simulink model "MR30Simulinknodos"  (R2013a)
settings: Solver=ode23tb  StartTime=0.0  StopTime=10.0  RelTol=1e-3
libraries: powerlib x200
(part 2 of 2)

== system MR30Simulinknodos/BUSstep B25 ==
  " (RL1)/2" : powerlib/Elements/Series RLC Branch  LConnTagsString=__new0  RConnTagsString=__new0  BranchType=R  Resistance=1.560804/2  Inductance=1e-3  SetiL0=off  InitialCurrent=0  Capacitance=1e-6  Setx0=off  InitialVoltage=0  Measurements=None
  " (RL3)/2" : powerlib/Elements/Series RLC Branch  LConnTagsString=__new0  RConnTagsString=__new0  BranchType=R  Resistance=3.632832/2  Inductance=1e-3  SetiL0=off  InitialCurrent=0  Capacitance=1e-6  Setx0=off  InitialVoltage=0  Measurements=None
  " (RLn)/2" : powerlib/Elements/Series RLC Branch  LConnTagsString=__new0  RConnTagsString=__new0  BranchType=R  Resistance=2.69178/2  Inductance=1e-3  SetiL0=off  InitialCurrent=0  Capacitance=1e-6  Setx0=off  InitialVoltage=0  Measurements=None
  Ground : powerlib/Elements/Ground  LConnTagsString=a
  Voltage Measurement : powerlib/Measurements/Voltage Measurement  PhasorSimulation=off  OutputType=Complex  PSBequivalent=0
  L35 : PMIOPort  Port=1  Side=Right
  L34 : PMIOPort  Port=2  Side=Right
  L33 : PMIOPort  Port=3  Side=Left
  VBUSstep : Outport
  wires:
  Voltage Measurement/1 -> VBUSstep/1
  connections:
  L33/RConn1 -- " (RLn)/2"/RConn1
  " (RL3)/2"/RConn1 -- " (RLn)/2"/LConn1 -- " (RL1)/2"/LConn1 -- Voltage Measurement/LConn1
  Ground/LConn1 -- Voltage Measurement/LConn2
  " (RL3)/2"/LConn1 -- L34/RConn1
  " (RL1)/2"/RConn1 -- L35/RConn1

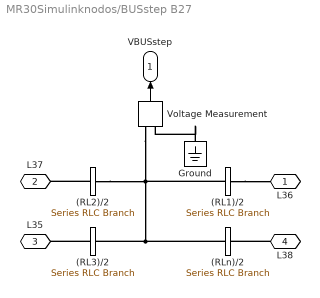
== system MR30Simulinknodos/BUSstep B27 ==
  " (RL1)/2" : powerlib/Elements/Series RLC Branch  LConnTagsString=__new0  RConnTagsString=__new0  BranchType=R  Resistance=5.65488/2  Inductance=1e-3  SetiL0=off  InitialCurrent=0  Capacitance=1e-6  Setx0=off  InitialVoltage=0  Measurements=None
  " (RL2)/2" : powerlib/Elements/Series RLC Branch  LConnTagsString=__new0  RConnTagsString=__new0  BranchType=R  Resistance=3.138744/2  Inductance=1e-3  SetiL0=off  InitialCurrent=0  Capacitance=1e-6  Setx0=off  InitialVoltage=0  Measurements=None
  " (RL3)/2" : powerlib/Elements/Series RLC Branch  LConnTagsString=__new0  RConnTagsString=__new0  BranchType=R  Resistance=1.560804/2  Inductance=1e-3  SetiL0=off  InitialCurrent=0  Capacitance=1e-6  Setx0=off  InitialVoltage=0  Measurements=None
  " (RLn)/2" : powerlib/Elements/Series RLC Branch  LConnTagsString=__new0  RConnTagsString=__new0  BranchType=R  Resistance=4.572456/2  Inductance=1e-3  SetiL0=off  InitialCurrent=0  Capacitance=1e-6  Setx0=off  InitialVoltage=0  Measurements=None
  Ground : powerlib/Elements/Ground  LConnTagsString=a
  Voltage Measurement : powerlib/Measurements/Voltage Measurement  PhasorSimulation=off  OutputType=Complex  PSBequivalent=0
  L36 : PMIOPort  Port=1  Side=Right
  L37 : PMIOPort  Port=2  Side=Left
  L35 : PMIOPort  Port=3  Side=Right
  L38 : PMIOPort  Port=4  Side=Left
  VBUSstep : Outport
  wires:
  Voltage Measurement/1 -> VBUSstep/1
  connections:
  " (RL1)/2"/RConn1 -- L36/RConn1
  " (RL3)/2"/LConn1 -- L35/RConn1
  " (RL2)/2"/LConn1 -- L37/RConn1
  Ground/LConn1 -- Voltage Measurement/LConn2
  Voltage Measurement/LConn1 -- " (RL2)/2"/RConn1 -- " (RL1)/2"/LConn1 -- " (RLn)/2"/LConn1 -- " (RL3)/2"/RConn1
  L38/RConn1 -- " (RLn)/2"/RConn1

== system MR30Simulinknodos/BUSstep B28 ==
  " (RL1)/2" : powerlib/Elements/Series RLC Branch  LConnTagsString=__new0  RConnTagsString=__new0  BranchType=R  Resistance=0.908208/2  Inductance=1e-3  SetiL0=off  InitialCurrent=0  Capacitance=1e-6  Setx0=off  InitialVoltage=0  Measurements=None
  " (RL2)/2" : powerlib/Elements/Series RLC Branch  LConnTagsString=__new0  RConnTagsString=__new0  BranchType=R  Resistance=5.65488/2  Inductance=1e-3  SetiL0=off  InitialCurrent=0  Capacitance=1e-6  Setx0=off  InitialVoltage=0  Measurements=None
  " (RL3)/2" : powerlib/Elements/Series RLC Branch  LConnTagsString=__new0  RConnTagsString=__new0  BranchType=R  Resistance=2.41332/2  Inductance=1e-3  SetiL0=off  InitialCurrent=0  Capacitance=1e-6  Setx0=off  InitialVoltage=0  Measurements=None
  Ground : powerlib/Elements/Ground  LConnTagsString=a
  Voltage Measurement : powerlib/Measurements/Voltage Measurement  PhasorSimulation=off  OutputType=Complex  PSBequivalent=0
  L40 : PMIOPort  Port=1  Side=Right
  L36 : PMIOPort  Port=2  Side=Left
  L41 : PMIOPort  Port=3  Side=Right
  VBUSstep : Outport
  wires:
  Voltage Measurement/1 -> VBUSstep/1
  connections:
  " (RL3)/2"/RConn1 -- " (RL1)/2"/LConn1 -- " (RL2)/2"/RConn1 -- Voltage Measurement/LConn1
  Ground/LConn1 -- Voltage Measurement/LConn2
  " (RL2)/2"/LConn1 -- L36/RConn1
  " (RL3)/2"/LConn1 -- L41/RConn1
  " (RL1)/2"/RConn1 -- L40/RConn1

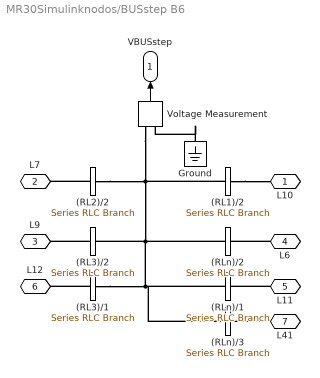
== system MR30Simulinknodos/BUSstep B6 ==
  " (RL1)/2" : powerlib/Elements/Series RLC Branch  LConnTagsString=__new0  RConnTagsString=__new0  BranchType=R  Resistance=.17136/2  Inductance=1e-3  SetiL0=off  InitialCurrent=0  Capacitance=1e-6  Setx0=off  InitialVoltage=0  Measurements=None
  " (RL2)/2" : powerlib/Elements/Series RLC Branch  LConnTagsString=__new0  RConnTagsString=__new0  BranchType=R  Resistance=0.169932/2  Inductance=1e-3  SetiL0=off  InitialCurrent=0  Capacitance=1e-6  Setx0=off  InitialVoltage=0  Measurements=None
  " (RL3)/1" : powerlib/Elements/Series RLC Branch  LConnTagsString=__new0  RConnTagsString=__new0  BranchType=R  Resistance=7.93968/2  Inductance=1e-3  SetiL0=off  InitialCurrent=0  Capacitance=1e-6  Setx0=off  InitialVoltage=0  Measurements=None
  " (RL3)/2" : powerlib/Elements/Series RLC Branch  LConnTagsString=__new0  RConnTagsString=__new0  BranchType=R  Resistance=.381276/2  Inductance=1e-3  SetiL0=off  InitialCurrent=0  Capacitance=1e-6  Setx0=off  InitialVoltage=0  Measurements=None
  " (RLn)/1" : powerlib/Elements/Series RLC Branch  LConnTagsString=__new0  RConnTagsString=__new0  BranchType=R  Resistance=2.97024/2  Inductance=1e-3  SetiL0=off  InitialCurrent=0  Capacitance=1e-6  Setx0=off  InitialVoltage=0  Measurements=None
  " (RLn)/2" : powerlib/Elements/Series RLC Branch  LConnTagsString=__new0  RConnTagsString=__new0  BranchType=R  Resistance=.829668/2  Inductance=1e-3  SetiL0=off  InitialCurrent=0  Capacitance=1e-6  Setx0=off  InitialVoltage=0  Measurements=None
  " (RLn)/3" : powerlib/Elements/Series RLC Branch  LConnTagsString=__new0  RConnTagsString=__new0  BranchType=R  Resistance=2.41332/2  Inductance=1e-3  SetiL0=off  InitialCurrent=0  Capacitance=1e-6  Setx0=off  InitialVoltage=0  Measurements=None
  Ground : powerlib/Elements/Ground  LConnTagsString=a
  Voltage Measurement : powerlib/Measurements/Voltage Measurement  PhasorSimulation=off  OutputType=Complex  PSBequivalent=0
  L10 : PMIOPort  Port=1  Side=Right
  L7 : PMIOPort  Port=2  Side=Left
  L9 : PMIOPort  Port=3  Side=Right
  L6 : PMIOPort  Port=4  Side=Left
  L11 : PMIOPort  Port=5  Side=Left
  L12 : PMIOPort  Port=6  Side=Right
  L41 : PMIOPort  Port=7  Side=Left
  VBUSstep : Outport
  wires:
  Voltage Measurement/1 -> VBUSstep/1
  connections:
  " (RL1)/2"/RConn1 -- L10/RConn1
  " (RL3)/2"/LConn1 -- L9/RConn1
  " (RL2)/2"/LConn1 -- L7/RConn1
  Ground/LConn1 -- Voltage Measurement/LConn2
  Voltage Measurement/LConn1 -- " (RL2)/2"/RConn1 -- " (RL1)/2"/LConn1 -- " (RLn)/3"/LConn1 -- " (RLn)/1"/LConn1 -- " (RL3)/1"/RConn1 -- " (RLn)/2"/LConn1 -- " (RL3)/2"/RConn1
  L6/RConn1 -- " (RLn)/2"/RConn1
  L11/RConn1 -- " (RLn)/1"/RConn1
  " (RL3)/1"/LConn1 -- L12/RConn1
  L41/RConn1 -- " (RLn)/3"/RConn1

== system MR30Simulinknodos/BUSstep B9 ==
  " (RL1)/2" : powerlib/Elements/Series RLC Branch  LConnTagsString=__new0  RConnTagsString=__new0  BranchType=R  Resistance=1.5708/2  Inductance=1e-3  SetiL0=off  InitialCurrent=0  Capacitance=1e-6  Setx0=off  InitialVoltage=0  Measurements=None
  " (RL2)/2" : powerlib/Elements/Series RLC Branch  LConnTagsString=__new0  RConnTagsString=__new0  BranchType=R  Resistance=2.97024/2  Inductance=1e-3  SetiL0=off  InitialCurrent=0  Capacitance=1e-6  Setx0=off  InitialVoltage=0  Measurements=None
  " (RLn)/2" : powerlib/Elements/Series RLC Branch  LConnTagsString=__new0  RConnTagsString=__new0  BranchType=R  Resistance=2.97024/2  Inductance=1e-3  SetiL0=off  InitialCurrent=0  Capacitance=1e-6  Setx0=off  InitialVoltage=0  Measurements=None
  Ground : powerlib/Elements/Ground  LConnTagsString=a
  Voltage Measurement : powerlib/Measurements/Voltage Measurement  PhasorSimulation=off  OutputType=Complex  PSBequivalent=0
  L14 : PMIOPort  Port=1  Side=Right
  L13 : PMIOPort  Port=2  Side=Left
  L11 : PMIOPort  Port=3  Side=Left
  VBUSstep : Outport
  wires:
  Voltage Measurement/1 -> VBUSstep/1
  connections:
  L11/RConn1 -- " (RLn)/2"/RConn1
  " (RLn)/2"/LConn1 -- " (RL1)/2"/LConn1 -- " (RL2)/2"/RConn1 -- Voltage Measurement/LConn1
  Ground/LConn1 -- Voltage Measurement/LConn2
  " (RL2)/2"/LConn1 -- L13/RConn1
  " (RL1)/2"/RConn1 -- L14/RConn1

== system MR30Simulinknodos/DG1 ==
  VBUS1 : Inport
  IBUS1 : Inport  Port=2
  DroopDG1 : Subsystem
  G1 : powerlib/Electrical Sources/Controlled Voltage Source  Initialize=on  Source_Type=DC  Amplitude=1000  Phase=0  Frequency=0  Measurements=None
  Ground : powerlib/Elements/Ground  LConnTagsString=a
  DG1+ : PMIOPort  Port=1  Side=Right
  DG1- : PMIOPort  Port=2  Side=Right
  PBUS1 : Outport
  wires:
  DroopDG1/2(PDG1) -> PBUS1/1
  IBUS1/1 -> DroopDG1/2(IG1)
  VBUS1/1 -> DroopDG1/1(VG1)
  DroopDG1/1(Vdroop1) -> G1/1
  connections:
  G1/LConn1 -- DG1-/RConn1 -- Ground/LConn1
  DG1+/RConn1 -- G1/RConn1

== system MR30Simulinknodos/DG2 ==
  VBUS2 : Inport
  IBUS2 : Inport  Port=2
  DroopDG1 : Subsystem
  G1 : powerlib/Electrical Sources/Controlled Voltage Source  Initialize=on  Source_Type=DC  Amplitude=1000  Phase=0  Frequency=0  Measurements=None
  Ground : powerlib/Elements/Ground  LConnTagsString=a
  DG2+ : PMIOPort  Port=1  Side=Right
  DG2- : PMIOPort  Port=2  Side=Right
  PBUS2 : Outport
  wires:
  VBUS2/1 -> DroopDG1/1(VG1)
  IBUS2/1 -> DroopDG1/2(IG1)
  DroopDG1/2(PDG1) -> PBUS2/1
  DroopDG1/1(Vdroop1) -> G1/1
  connections:
  DG2+/RConn1 -- G1/RConn1
  Ground/LConn1 -- DG2-/RConn1 -- G1/LConn1

== system MR30Simulinknodos/DG3 ==
  VBUS5 : Inport
  IBUS5 : Inport  Port=2
  DroopDG1 : Subsystem
  G1 : powerlib/Electrical Sources/Controlled Voltage Source  Initialize=on  Source_Type=DC  Amplitude=1000  Phase=0  Frequency=0  Measurements=None
  Ground : powerlib/Elements/Ground  LConnTagsString=a
  DG3+ : PMIOPort  Port=1  Side=Right
  DG3- : PMIOPort  Port=2  Side=Right
  PBUS5 : Outport
  wires:
  DroopDG1/2(PDG1) -> PBUS5/1
  IBUS5/1 -> DroopDG1/2(IG1)
  VBUS5/1 -> DroopDG1/1(VG1)
  DroopDG1/1(Vdroop1) -> G1/1
  connections:
  G1/LConn1 -- DG3-/RConn1 -- Ground/LConn1
  DG3+/RConn1 -- G1/RConn1

== system MR30Simulinknodos/DG4 ==
  VBUS8 : Inport
  IBUS8 : Inport  Port=2
  DroopDG1 : Subsystem
  G1 : powerlib/Electrical Sources/Controlled Voltage Source  Initialize=on  Source_Type=DC  Amplitude=1000  Phase=0  Frequency=0  Measurements=None
  Ground : powerlib/Elements/Ground  LConnTagsString=a
  DG4+ : PMIOPort  Port=1  Side=Right
  DG4- : PMIOPort  Port=2  Side=Right
  PBUS8 : Outport
  wires:
  VBUS8/1 -> DroopDG1/1(VG1)
  IBUS8/1 -> DroopDG1/2(IG1)
  DroopDG1/2(PDG1) -> PBUS8/1
  DroopDG1/1(Vdroop1) -> G1/1
  connections:
  DG4+/RConn1 -- G1/RConn1
  Ground/LConn1 -- DG4-/RConn1 -- G1/LConn1

== system MR30Simulinknodos/DG5 ==
  VBUS11 : Inport
  IBUS11 : Inport  Port=2
  DroopDG1 : Subsystem
  G1 : powerlib/Electrical Sources/Controlled Voltage Source  Initialize=on  Source_Type=DC  Amplitude=1000  Phase=0  Frequency=0  Measurements=None
  Ground : powerlib/Elements/Ground  LConnTagsString=a
  DG5+ : PMIOPort  Port=1  Side=Right
  DG5- : PMIOPort  Port=2  Side=Right
  PBUS11 : Outport
  wires:
  VBUS11/1 -> DroopDG1/1(VG1)
  IBUS11/1 -> DroopDG1/2(IG1)
  DroopDG1/2(PDG1) -> PBUS11/1
  DroopDG1/1(Vdroop1) -> G1/1
  connections:
  DG5+/RConn1 -- G1/RConn1
  Ground/LConn1 -- DG5-/RConn1 -- G1/LConn1

== system MR30Simulinknodos/DG6 ==
  VBUS13 : Inport
  IBUS13 : Inport  Port=2
  DroopDG1 : Subsystem
  G1 : powerlib/Electrical Sources/Controlled Voltage Source  Initialize=on  Source_Type=DC  Amplitude=1000  Phase=0  Frequency=0  Measurements=None
  Ground : powerlib/Elements/Ground  LConnTagsString=a
  DG6+ : PMIOPort  Port=1  Side=Right
  DG6- : PMIOPort  Port=2  Side=Right
  PBUS13 : Outport
  wires:
  DroopDG1/2(PDG1) -> PBUS13/1
  IBUS13/1 -> DroopDG1/2(IG1)
  VBUS13/1 -> DroopDG1/1(VG1)
  DroopDG1/1(Vdroop1) -> G1/1
  connections:
  G1/LConn1 -- DG6-/RConn1 -- Ground/LConn1
  DG6+/RConn1 -- G1/RConn1

== system MR30Simulinknodos/Load1 ==
  VBUSc : Inport
  Constant4 : Constant  Value=21700
  Controlled Current Source : powerlib/Electrical Sources/Controlled Current Source  Initialize=off  Source_Type=DC  Amplitude=0  Phase=0  Frequency=0  Measurements=None
  Divide2 : Product  Inputs=*/
  Ground3 : powerlib/Elements/Ground  LConnTagsString=a
  Load1+ : PMIOPort  Port=1  Side=Left
  Load1- : PMIOPort  Port=2  Side=Left
  wires:
  Constant4/1 -> Divide2/1
  Divide2/1 -> Controlled Current Source/1
  VBUSc/1 -> Divide2/2
  connections:
  Controlled Current Source/RConn1 -- Load1-/RConn1 -- Ground3/LConn1
  Controlled Current Source/LConn1 -- Load1+/RConn1

== system MR30Simulinknodos/Load10 ==
  VBUSc : Inport
  Constant4 : Constant  Value=8200
  Controlled Current Source : powerlib/Electrical Sources/Controlled Current Source  Initialize=off  Source_Type=DC  Amplitude=0  Phase=0  Frequency=0  Measurements=None
  Divide2 : Product  Inputs=*/
  Ground3 : powerlib/Elements/Ground  LConnTagsString=a
  Load1+ : PMIOPort  Port=1  Side=Left
  Load1- : PMIOPort  Port=2  Side=Left
  wires:
  VBUSc/1 -> Divide2/2
  Divide2/1 -> Controlled Current Source/1
  Constant4/1 -> Divide2/1
  connections:
  Controlled Current Source/LConn1 -- Load1+/RConn1
  Ground3/LConn1 -- Load1-/RConn1 -- Controlled Current Source/RConn1

== system MR30Simulinknodos/Load11 ==
  VBUSc : Inport
  Constant4 : Constant  Value=3500
  Controlled Current Source : powerlib/Electrical Sources/Controlled Current Source  Initialize=off  Source_Type=DC  Amplitude=0  Phase=0  Frequency=0  Measurements=None
  Divide2 : Product  Inputs=*/
  Ground3 : powerlib/Elements/Ground  LConnTagsString=a
  Load1+ : PMIOPort  Port=1  Side=Left
  Load1- : PMIOPort  Port=2  Side=Left
  wires:
  Constant4/1 -> Divide2/1
  Divide2/1 -> Controlled Current Source/1
  VBUSc/1 -> Divide2/2
  connections:
  Controlled Current Source/RConn1 -- Load1-/RConn1 -- Ground3/LConn1
  Controlled Current Source/LConn1 -- Load1+/RConn1

== system MR30Simulinknodos/Load12 ==
  VBUSc : Inport
  Constant4 : Constant  Value=9000
  Controlled Current Source : powerlib/Electrical Sources/Controlled Current Source  Initialize=off  Source_Type=DC  Amplitude=0  Phase=0  Frequency=0  Measurements=None
  Divide2 : Product  Inputs=*/
  Ground3 : powerlib/Elements/Ground  LConnTagsString=a
  Load1+ : PMIOPort  Port=1  Side=Left
  Load1- : PMIOPort  Port=2  Side=Left
  wires:
  VBUSc/1 -> Divide2/2
  Divide2/1 -> Controlled Current Source/1
  Constant4/1 -> Divide2/1
  connections:
  Controlled Current Source/LConn1 -- Load1+/RConn1
  Ground3/LConn1 -- Load1-/RConn1 -- Controlled Current Source/RConn1

== system MR30Simulinknodos/Load13 ==
  VBUSc : Inport
  Constant4 : Constant  Value=3200
  Controlled Current Source : powerlib/Electrical Sources/Controlled Current Source  Initialize=off  Source_Type=DC  Amplitude=0  Phase=0  Frequency=0  Measurements=None
  Divide2 : Product  Inputs=*/
  Ground3 : powerlib/Elements/Ground  LConnTagsString=a
  Load1+ : PMIOPort  Port=1  Side=Left
  Load1- : PMIOPort  Port=2  Side=Left
  wires:
  Constant4/1 -> Divide2/1
  Divide2/1 -> Controlled Current Source/1
  VBUSc/1 -> Divide2/2
  connections:
  Controlled Current Source/RConn1 -- Load1-/RConn1 -- Ground3/LConn1
  Controlled Current Source/LConn1 -- Load1+/RConn1

== system MR30Simulinknodos/Load14 ==
  VBUSc : Inport
  Constant4 : Constant  Value=9500
  Controlled Current Source : powerlib/Electrical Sources/Controlled Current Source  Initialize=off  Source_Type=DC  Amplitude=0  Phase=0  Frequency=0  Measurements=None
  Divide2 : Product  Inputs=*/
  Ground3 : powerlib/Elements/Ground  LConnTagsString=a
  Load1+ : PMIOPort  Port=1  Side=Left
  Load1- : PMIOPort  Port=2  Side=Left
  wires:
  VBUSc/1 -> Divide2/2
  Divide2/1 -> Controlled Current Source/1
  Constant4/1 -> Divide2/1
  connections:
  Controlled Current Source/LConn1 -- Load1+/RConn1
  Ground3/LConn1 -- Load1-/RConn1 -- Controlled Current Source/RConn1

== system MR30Simulinknodos/Load15 ==
  VBUSc : Inport
  Constant4 : Constant  Value=2200
  Controlled Current Source : powerlib/Electrical Sources/Controlled Current Source  Initialize=off  Source_Type=DC  Amplitude=0  Phase=0  Frequency=0  Measurements=None
  Divide2 : Product  Inputs=*/
  Ground3 : powerlib/Elements/Ground  LConnTagsString=a
  Load1+ : PMIOPort  Port=1  Side=Left
  Load1- : PMIOPort  Port=2  Side=Left
  wires:
  Constant4/1 -> Divide2/1
  Divide2/1 -> Controlled Current Source/1
  VBUSc/1 -> Divide2/2
  connections:
  Controlled Current Source/RConn1 -- Load1-/RConn1 -- Ground3/LConn1
  Controlled Current Source/LConn1 -- Load1+/RConn1

== system MR30Simulinknodos/Load16 ==
  VBUSc : Inport
  Constant4 : Constant  Value=17500
  Controlled Current Source : powerlib/Electrical Sources/Controlled Current Source  Initialize=off  Source_Type=DC  Amplitude=0  Phase=0  Frequency=0  Measurements=None
  Divide2 : Product  Inputs=*/
  Ground3 : powerlib/Elements/Ground  LConnTagsString=a
  Load1+ : PMIOPort  Port=1  Side=Left
  Load1- : PMIOPort  Port=2  Side=Left
  wires:
  Constant4/1 -> Divide2/1
  Divide2/1 -> Controlled Current Source/1
  VBUSc/1 -> Divide2/2
  connections:
  Controlled Current Source/RConn1 -- Load1-/RConn1 -- Ground3/LConn1
  Controlled Current Source/LConn1 -- Load1+/RConn1

== system MR30Simulinknodos/Load17 ==
  VBUSc : Inport
  Constant4 : Constant  Value=3200
  Controlled Current Source : powerlib/Electrical Sources/Controlled Current Source  Initialize=off  Source_Type=DC  Amplitude=0  Phase=0  Frequency=0  Measurements=None
  Divide2 : Product  Inputs=*/
  Ground3 : powerlib/Elements/Ground  LConnTagsString=a
  Load1+ : PMIOPort  Port=1  Side=Left
  Load1- : PMIOPort  Port=2  Side=Left
  wires:
  Constant4/1 -> Divide2/1
  Divide2/1 -> Controlled Current Source/1
  VBUSc/1 -> Divide2/2
  connections:
  Controlled Current Source/RConn1 -- Load1-/RConn1 -- Ground3/LConn1
  Controlled Current Source/LConn1 -- Load1+/RConn1

== system MR30Simulinknodos/Load18 ==
  VBUSc : Inport
  Constant4 : Constant  Value=8700
  Controlled Current Source : powerlib/Electrical Sources/Controlled Current Source  Initialize=off  Source_Type=DC  Amplitude=0  Phase=0  Frequency=0  Measurements=None
  Divide2 : Product  Inputs=*/
  Ground3 : powerlib/Elements/Ground  LConnTagsString=a
  Load1+ : PMIOPort  Port=1  Side=Left
  Load1- : PMIOPort  Port=2  Side=Left
  wires:
  VBUSc/1 -> Divide2/2
  Divide2/1 -> Controlled Current Source/1
  Constant4/1 -> Divide2/1
  connections:
  Controlled Current Source/LConn1 -- Load1+/RConn1
  Ground3/LConn1 -- Load1-/RConn1 -- Controlled Current Source/RConn1

== system MR30Simulinknodos/Load19 ==
  VBUSc : Inport
  Constant4 : Constant  Value=3500
  Controlled Current Source : powerlib/Electrical Sources/Controlled Current Source  Initialize=off  Source_Type=DC  Amplitude=0  Phase=0  Frequency=0  Measurements=None
  Divide2 : Product  Inputs=*/
  Ground3 : powerlib/Elements/Ground  LConnTagsString=a
  Load1+ : PMIOPort  Port=1  Side=Left
  Load1- : PMIOPort  Port=2  Side=Left
  wires:
  VBUSc/1 -> Divide2/2
  Divide2/1 -> Controlled Current Source/1
  Constant4/1 -> Divide2/1
  connections:
  Controlled Current Source/LConn1 -- Load1+/RConn1
  Ground3/LConn1 -- Load1-/RConn1 -- Controlled Current Source/RConn1

== system MR30Simulinknodos/Load2 ==
  VBUSc : Inport
  Constant4 : Constant  Value=2400
  Controlled Current Source : powerlib/Electrical Sources/Controlled Current Source  Initialize=off  Source_Type=DC  Amplitude=0  Phase=0  Frequency=0  Measurements=None
  Divide2 : Product  Inputs=*/
  Ground3 : powerlib/Elements/Ground  LConnTagsString=a
  Load1+ : PMIOPort  Port=1  Side=Left
  Load1- : PMIOPort  Port=2  Side=Left
  wires:
  VBUSc/1 -> Divide2/2
  Divide2/1 -> Controlled Current Source/1
  Constant4/1 -> Divide2/1
  connections:
  Controlled Current Source/LConn1 -- Load1+/RConn1
  Ground3/LConn1 -- Load1-/RConn1 -- Controlled Current Source/RConn1

== system MR30Simulinknodos/Load20 ==
  VBUSc : Inport
  Constant4 : Constant  Value=2400
  Controlled Current Source : powerlib/Electrical Sources/Controlled Current Source  Initialize=off  Source_Type=DC  Amplitude=0  Phase=0  Frequency=0  Measurements=None
  Divide2 : Product  Inputs=*/
  Ground3 : powerlib/Elements/Ground  LConnTagsString=a
  Load1+ : PMIOPort  Port=1  Side=Left
  Load1- : PMIOPort  Port=2  Side=Left
  wires:
  Constant4/1 -> Divide2/1
  Divide2/1 -> Controlled Current Source/1
  VBUSc/1 -> Divide2/2
  connections:
  Controlled Current Source/RConn1 -- Load1-/RConn1 -- Ground3/LConn1
  Controlled Current Source/LConn1 -- Load1+/RConn1

== system MR30Simulinknodos/Load21 ==
  VBUSc : Inport
  Constant4 : Constant  Value=10600
  Controlled Current Source : powerlib/Electrical Sources/Controlled Current Source  Initialize=off  Source_Type=DC  Amplitude=0  Phase=0  Frequency=0  Measurements=None
  Divide2 : Product  Inputs=*/
  Ground3 : powerlib/Elements/Ground  LConnTagsString=a
  Load1+ : PMIOPort  Port=1  Side=Left
  Load1- : PMIOPort  Port=2  Side=Left
  wires:
  VBUSc/1 -> Divide2/2
  Divide2/1 -> Controlled Current Source/1
  Constant4/1 -> Divide2/1
  connections:
  Controlled Current Source/LConn1 -- Load1+/RConn1
  Ground3/LConn1 -- Load1-/RConn1 -- Controlled Current Source/RConn1

== system MR30Simulinknodos/Load3 ==
  VBUSc : Inport
  Constant4 : Constant  Value=7600
  Controlled Current Source : powerlib/Electrical Sources/Controlled Current Source  Initialize=off  Source_Type=DC  Amplitude=0  Phase=0  Frequency=0  Measurements=None
  Divide2 : Product  Inputs=*/
  Ground3 : powerlib/Elements/Ground  LConnTagsString=a
  Load1+ : PMIOPort  Port=1  Side=Left
  Load1- : PMIOPort  Port=2  Side=Left
  wires:
  Constant4/1 -> Divide2/1
  Divide2/1 -> Controlled Current Source/1
  VBUSc/1 -> Divide2/2
  connections:
  Controlled Current Source/RConn1 -- Load1-/RConn1 -- Ground3/LConn1
  Controlled Current Source/LConn1 -- Load1+/RConn1

== system MR30Simulinknodos/Load4 ==
  VBUSc : Inport
  Constant4 : Constant  Value=19000
  Controlled Current Source : powerlib/Electrical Sources/Controlled Current Source  Initialize=off  Source_Type=DC  Amplitude=0  Phase=0  Frequency=0  Measurements=None
  Divide2 : Product  Inputs=*/
  Ground3 : powerlib/Elements/Ground  LConnTagsString=a
  Load1+ : PMIOPort  Port=1  Side=Left
  Load1- : PMIOPort  Port=2  Side=Left
  wires:
  VBUSc/1 -> Divide2/2
  Divide2/1 -> Controlled Current Source/1
  Constant4/1 -> Divide2/1
  connections:
  Controlled Current Source/LConn1 -- Load1+/RConn1
  Ground3/LConn1 -- Load1-/RConn1 -- Controlled Current Source/RConn1

== system MR30Simulinknodos/Load5 ==
  VBUSc : Inport
  Constant4 : Constant  Value=22800
  Controlled Current Source : powerlib/Electrical Sources/Controlled Current Source  Initialize=off  Source_Type=DC  Amplitude=0  Phase=0  Frequency=0  Measurements=None
  Divide2 : Product  Inputs=*/
  Ground3 : powerlib/Elements/Ground  LConnTagsString=a
  Load1+ : PMIOPort  Port=1  Side=Left
  Load1- : PMIOPort  Port=2  Side=Left
  wires:
  VBUSc/1 -> Divide2/2
  Divide2/1 -> Controlled Current Source/1
  Constant4/1 -> Divide2/1
  connections:
  Controlled Current Source/LConn1 -- Load1+/RConn1
  Ground3/LConn1 -- Load1-/RConn1 -- Controlled Current Source/RConn1

== system MR30Simulinknodos/Load6 ==
  VBUSc : Inport
  Constant4 : Constant  Value=15000
  Controlled Current Source : powerlib/Electrical Sources/Controlled Current Source  Initialize=off  Source_Type=DC  Amplitude=0  Phase=0  Frequency=0  Measurements=None
  Divide2 : Product  Inputs=*/
  Ground3 : powerlib/Elements/Ground  LConnTagsString=a
  Load1+ : PMIOPort  Port=1  Side=Left
  Load1- : PMIOPort  Port=2  Side=Left
  wires:
  Constant4/1 -> Divide2/1
  Divide2/1 -> Controlled Current Source/1
  VBUSc/1 -> Divide2/2
  connections:
  Controlled Current Source/RConn1 -- Load1-/RConn1 -- Ground3/LConn1
  Controlled Current Source/LConn1 -- Load1+/RConn1

== system MR30Simulinknodos/Load7 ==
  VBUSc : Inport
  Constant4 : Constant  Value=5800
  Controlled Current Source : powerlib/Electrical Sources/Controlled Current Source  Initialize=off  Source_Type=DC  Amplitude=0  Phase=0  Frequency=0  Measurements=None
  Divide2 : Product  Inputs=*/
  Ground3 : powerlib/Elements/Ground  LConnTagsString=a
  Load1+ : PMIOPort  Port=1  Side=Left
  Load1- : PMIOPort  Port=2  Side=Left
  wires:
  Constant4/1 -> Divide2/1
  Divide2/1 -> Controlled Current Source/1
  VBUSc/1 -> Divide2/2
  connections:
  Controlled Current Source/RConn1 -- Load1-/RConn1 -- Ground3/LConn1
  Controlled Current Source/LConn1 -- Load1+/RConn1

== system MR30Simulinknodos/Load8 ==
  VBUSc : Inport
  Constant4 : Constant  Value=11200
  Controlled Current Source : powerlib/Electrical Sources/Controlled Current Source  Initialize=off  Source_Type=DC  Amplitude=0  Phase=0  Frequency=0  Measurements=None
  Divide2 : Product  Inputs=*/
  Ground3 : powerlib/Elements/Ground  LConnTagsString=a
  Load1+ : PMIOPort  Port=1  Side=Left
  Load1- : PMIOPort  Port=2  Side=Left
  wires:
  VBUSc/1 -> Divide2/2
  Divide2/1 -> Controlled Current Source/1
  Constant4/1 -> Divide2/1
  connections:
  Controlled Current Source/LConn1 -- Load1+/RConn1
  Ground3/LConn1 -- Load1-/RConn1 -- Controlled Current Source/RConn1

== system MR30Simulinknodos/Load9 ==
  VBUSc : Inport
  Constant4 : Constant  Value=6200
  Controlled Current Source : powerlib/Electrical Sources/Controlled Current Source  Initialize=off  Source_Type=DC  Amplitude=0  Phase=0  Frequency=0  Measurements=None
  Divide2 : Product  Inputs=*/
  Ground3 : powerlib/Elements/Ground  LConnTagsString=a
  Load1+ : PMIOPort  Port=1  Side=Left
  Load1- : PMIOPort  Port=2  Side=Left
  wires:
  Constant4/1 -> Divide2/1
  Divide2/1 -> Controlled Current Source/1
  VBUSc/1 -> Divide2/2
  connections:
  Controlled Current Source/RConn1 -- Load1-/RConn1 -- Ground3/LConn1
  Controlled Current Source/LConn1 -- Load1+/RConn1

== system MR30Simulinknodos/DG1/DroopDG1 ==
  VG1 : Inport
  IG1 : Inport  Port=2
  Constant : Constant  Value=1000
  Constant1 : Constant  Value=0.625
  Divide : Product  Inputs=**/
  Product : Product
  Sum : Sum  Inputs=+-|
  Vdroop1 : Outport
  PDG1 : Outport  Port=2
  wires:
  Constant1/1 -> Divide/1
  IG1/1 -> Product/2
  Constant/1 -> Sum/1
  Sum/1 -> Vdroop1/1
  Divide/1 -> Sum/2
  VG1/1 -> Product/1, Divide/3
  Product/1 -> Divide/2, PDG1/1

== system MR30Simulinknodos/DG2/DroopDG1 ==
  VG1 : Inport
  IG1 : Inport  Port=2
  Constant : Constant  Value=1000
  Constant1 : Constant  Value=1.25
  Divide : Product  Inputs=**/
  Product : Product
  Sum : Sum  Inputs=+-|
  Vdroop1 : Outport
  PDG1 : Outport  Port=2
  wires:
  Product/1 -> PDG1/1, Divide/2
  VG1/1 -> Divide/3, Product/1
  Divide/1 -> Sum/2
  Sum/1 -> Vdroop1/1
  Constant/1 -> Sum/1
  IG1/1 -> Product/2
  Constant1/1 -> Divide/1

== system MR30Simulinknodos/DG3/DroopDG1 ==
  VG1 : Inport
  IG1 : Inport  Port=2
  Constant : Constant  Value=1000
  Constant1 : Constant  Value=1.351
  Divide : Product  Inputs=**/
  Product : Product
  Sum : Sum  Inputs=+-|
  Vdroop1 : Outport
  PDG1 : Outport  Port=2
  wires:
  Constant1/1 -> Divide/1
  IG1/1 -> Product/2
  Constant/1 -> Sum/1
  Sum/1 -> Vdroop1/1
  Divide/1 -> Sum/2
  VG1/1 -> Product/1, Divide/3
  Product/1 -> Divide/2, PDG1/1

== system MR30Simulinknodos/DG4/DroopDG1 ==
  VG1 : Inport
  IG1 : Inport  Port=2
  Constant : Constant  Value=1000
  Constant1 : Constant  Value=1.31578947
  Divide : Product  Inputs=**/
  Product : Product
  Sum : Sum  Inputs=+-|
  Vdroop1 : Outport
  PDG1 : Outport  Port=2
  wires:
  Product/1 -> PDG1/1, Divide/2
  VG1/1 -> Divide/3, Product/1
  Divide/1 -> Sum/2
  Sum/1 -> Vdroop1/1
  Constant/1 -> Sum/1
  IG1/1 -> Product/2
  Constant1/1 -> Divide/1

== system MR30Simulinknodos/DG5/DroopDG1 ==
  VG1 : Inport
  IG1 : Inport  Port=2
  Constant : Constant  Value=1000
  Constant1 : Constant  Value=1.11111
  Divide : Product  Inputs=**/
  Product : Product
  Sum : Sum  Inputs=+-|
  Vdroop1 : Outport
  PDG1 : Outport  Port=2
  wires:
  Product/1 -> PDG1/1, Divide/2
  VG1/1 -> Divide/3, Product/1
  Divide/1 -> Sum/2
  Sum/1 -> Vdroop1/1
  Constant/1 -> Sum/1
  IG1/1 -> Product/2
  Constant1/1 -> Divide/1

== system MR30Simulinknodos/DG6/DroopDG1 ==
  VG1 : Inport
  IG1 : Inport  Port=2
  Constant : Constant  Value=1000
  Constant1 : Constant  Value=1.282051
  Divide : Product  Inputs=**/
  Product : Product
  Sum : Sum  Inputs=+-|
  Vdroop1 : Outport
  PDG1 : Outport  Port=2
  wires:
  Constant1/1 -> Divide/1
  IG1/1 -> Product/2
  Constant/1 -> Sum/1
  Sum/1 -> Vdroop1/1
  Divide/1 -> Sum/2
  VG1/1 -> Product/1, Divide/3
  Product/1 -> Divide/2, PDG1/1
